simulink library "uavsimBlockset_quaternionAttitudeController"  (Simulink 8.0)
settings: Solver=ode45  StartTime=0.0  StopTime=10.0  RelTol=1e-3
undefined symbols (not defined in the file): aircraftLibraryData, DiscIntNeverNeededParam
libraries: aerolibutil x3, uavsimBlockset_Quaternion2Rotationvector x1
settings Model: Creator=mstolle  LastModifiedBy=j.bolting

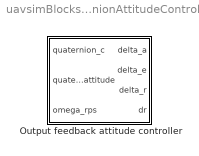
== system uavsimBlockset_quaternionAttitudeController ==
  Output feedback attitude controller : Subsystem  mask{mask_K=aircraftLibraryData.zagi.control.gains.K_attitude}
      mask prompts: mask_K "Feedback gain matrix K"

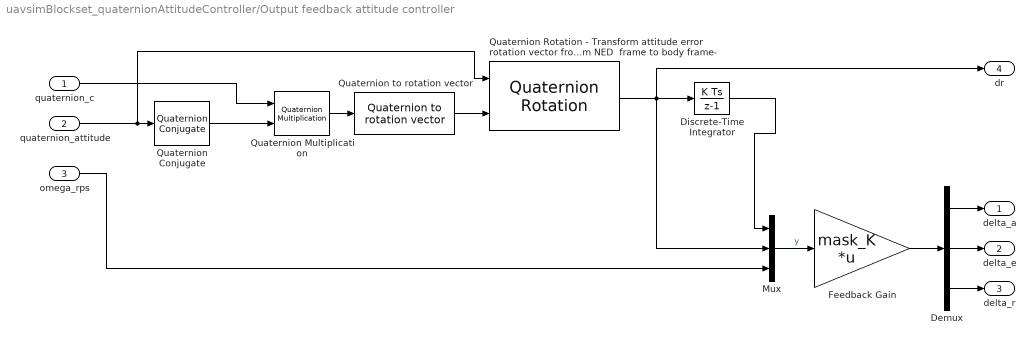
== system uavsimBlockset_quaternionAttitudeController/Output feedback attitude controller ==
  quaternion_c : Inport
  quaternion_attitude : Inport  Port=2
  omega_rps : Inport  Port=3
  Demux : Demux  Outputs=3
  Discrete-Time Integrator : DiscreteIntegrator  SampleTime=-1  ICPrevOutput=DiscIntNeverNeededParam  ICPrevScaledInput=DiscIntNeverNeededParam
  Feedback Gain : Gain  Gain=mask_K  Multiplication=Matrix(K*u)
  Mux : Mux  Inputs=3
  Quaternion to rotation vector : uavsimBlockset_Quaternion2Rotationvector/Quaternion to rotation vector
  Quaternion Conjugate : aerolibutil/Quaternion Conjugate
  Quaternion Multiplication : aerolibutil/Quaternion Multiplication
  Quaternion Rotation - Transform attitude error  rotation vector from NED  frame to body frame- : aerolibutil/Quaternion Rotation
  delta_a : Outport
  delta_e : Outport  Port=2
  delta_r : Outport  Port=3
  dr : Outport  Port=4
  wires:
  Quaternion Multiplication/1 -> Quaternion to rotation vector/1
  Discrete-Time Integrator/1 -> Mux/1
  quaternion_c/1 -> Quaternion Multiplication/1
  quaternion_attitude/1 -> Quaternion Rotation - Transform attitude error  rotation vector from NED  frame to body frame-/1, Quaternion Conjugate/1
  omega_rps/1 -> Mux/3
  Mux/1 -> Feedback Gain/1  "y"
  Feedback Gain/1 -> Demux/1
  Demux/3 -> delta_r/1
  Demux/2 -> delta_e/1
  Demux/1 -> delta_a/1
  Quaternion Conjugate/1 -> Quaternion Multiplication/2
  Quaternion to rotation vector/1 -> Quaternion Rotation - Transform attitude error  rotation vector from NED  frame to body frame-/2
  Quaternion Rotation - Transform attitude error  rotation vector from NED  frame to body frame-/1 -> dr/1, Mux/2, Discrete-Time Integrator/1
